simulink model "Praktikum02"  (R2023b)
settings: Solver=VariableStepAuto  StartTime=0.0  StopTime=10.0  RelTol=1e-3
model workspace (MAT data in the model file):
  M = 16
  Ts = 1e-06
undefined symbols (not defined in the file): doppler
libraries: commchan3 x8, commrflib2 x8, commdigbbndam3 x5, commsink2 x4, commrandsrc3 x1
settings Model: Creator=suttarar@hu-berlin.de

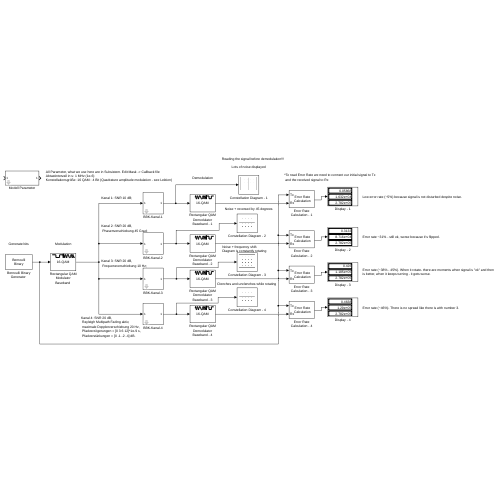
[thumbnail: Simulink's stored preview of the top-level diagram]
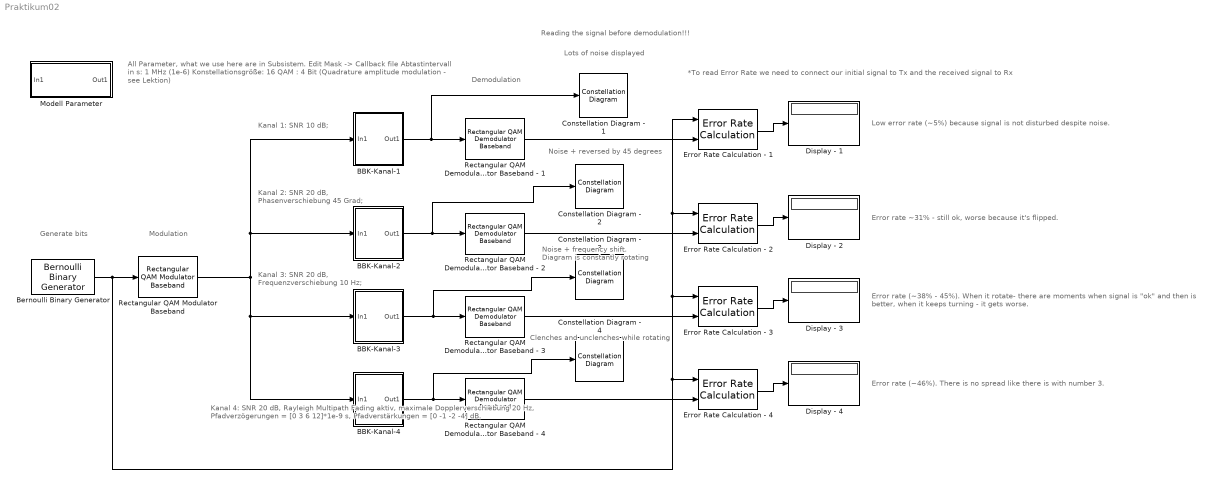
== system Praktikum02 ==
  note: Reading the signal before demodulation!!!
  note: *To read Error Rate we need to connect our initial signal to Tx
      |  and the received signal to Rx
  note: Error rate (~46%). There is no spread like there is with number 3.
  note: Clenches and unclenches while rotating
  note: Error rate (~38% - 45%). When it rotate- there are moments when signal is "ok" and then is better, when it keeps turning - it gets worse.
  note: Noise + frequency shift.
      | Diagram is constantly rotating
  note: Error rate ~31% - still ok, worse because it's flipped.
  note: Noise + reversed by 45 degrees
  note: Low error rate (~5%) because signal is not disturbed despite noise.
  note: Lots of noise displayed
  note: Kanal 4: SNR 20 dB,
      |  Rayleigh Multipath Fading aktiv,
      |  maximale Dopplerverschiebung 20 Hz,
      |  Pfadverzögerungen = [0 3 6 12]*1e-9 s,
      |  Pfadverstärkungen = [0 -1 -2 -4] dB.
  note: Kanal 3: SNR 20 dB,
      |  Frequenzverschiebung 10 Hz;
  note: Kanal 2: SNR 20 dB,
      |  Phasenverschiebung 45 Grad;
  note: Kanal 1: SNR 10 dB;
  note: Modulation
  note: Generate bits
  note: All Parameter, what we use here are in Subsistem. Edit Mask -> Callback file
      | Abtastintervall in s: 1 MHz (1e-6)
      | Konstellationsgröße: 16 QAM : 4 Bit (Quadrature amplitude modulation - see Lektion)
  note: Demodulation
  BBK-Kanal-1 : Subsystem  mask{MaxDoppler=20, PathDelays=[0 3 6 12]*1e-9, PathGains=[0 -1 -2 -4], EnableMultipath=0, PathLoss=0, FrequencyOffset=0, PhaseOffset=0, SNR=10}
      mask prompts: MaxDoppler "Dopplerverschiebung"; PathDelays "Pfadverzoergerungen"; PathGains "Pfadverstaerkungen"; EnableMultipath "SwitchBlock"; PathLoss "Pfadverlust"; FrequencyOffset "Frequenzverschiebung"; PhaseOffset "Phasenverschiebung"; SNR "AWG-Rauschen"
  BBK-Kanal-2 : Subsystem  mask{MaxDoppler=20, PathDelays=[0 3 6 12]*1e-9, PathGains=[0 -1 -2 -4], EnableMultipath=0, PathLoss=0, FrequencyOffset=0, PhaseOffset=45, SNR=20}
      mask prompts: MaxDoppler "Dopplerverschiebung"; PathDelays "Pfadverzoergerungen"; PathGains "Pfadverstaerkungen"; EnableMultipath "SwitchBlock"; PathLoss "Pfadverlust"; FrequencyOffset "Frequenzverschiebung"; PhaseOffset "Phasenverschiebung"; SNR "AWG-Rauschen"
  BBK-Kanal-3 : Subsystem  mask{MaxDoppler=20, PathDelays=[0 3 6 12]*1e-9, PathGains=[0 -1 -2 -4], EnableMultipath=0, PathLoss=0, FrequencyOffset=10, PhaseOffset=0, SNR=20}
      mask prompts: MaxDoppler "Dopplerverschiebung"; PathDelays "Pfadverzoergerungen"; PathGains "Pfadverstaerkungen"; EnableMultipath "SwitchBlock"; PathLoss "Pfadverlust"; FrequencyOffset "Frequenzverschiebung"; PhaseOffset "Phasenverschiebung"; SNR "AWG-Rauschen"
  BBK-Kanal-4 : Subsystem  mask{MaxDoppler=20, PathDelays=[0 3 6 12]*1e-9, PathGains=[0 -1 -2 -4], EnableMultipath=1, PathLoss=0, FrequencyOffset=0, PhaseOffset=0, SNR=20}
      mask prompts: MaxDoppler "Dopplerverschiebung"; PathDelays "Pfadverzoergerungen"; PathGains "Pfadverstaerkungen"; EnableMultipath "SwitchBlock"; PathLoss "Pfadverlust"; FrequencyOffset "Frequenzverschiebung"; PhaseOffset "Phasenverschiebung"; SNR "AWG-Rauschen"
  "Bernoulli Binary Generator " : commrandsrc3/Bernoulli Binary Generator  ProbabilityOfZero=0.5  SeedSource=Auto  Seed=0  SampleTime=Ts  SamplesPerFrame=log2(M)  OutputDataType=double  SimulateUsing=Interpreted execution
  Constellation Diagram - 1 : ConstellationDiagram  WindowPosition=[-8.000000,434.000000,600.000000,600.000000,]  Visible=on  ScopeFrameLocation=window  SymbolsToDisplaySource=Property  SymbolsToDisplay=500  XLimits=[-1.46,1.46]  YLimits=[-1.38,1.38]
  Constellation Diagram - 2 : ConstellationDiagram  WindowPosition=[602.000000,302.000000,600.000000,600.000000,]  Visible=on  ScopeFrameLocation=window  SymbolsToDisplaySource=Property  SymbolsToDisplay=500  ReferenceConstellation=QPSK  XLimits=[-1.46,1.46]  YLimits=[-1.38,1.38]
  Constellation Diagram - 3 : ConstellationDiagram  WindowPosition=[-15.000000,-148.000000,600.000000,600.000000,]  Visible=on  ScopeFrameLocation=window  SymbolsToDisplaySource=Property  SymbolsToDisplay=500  XLimits=[-1.46,1.46]  YLimits=[-1.38,1.38]
  Constellation Diagram - 4 : ConstellationDiagram  WindowPosition=[632.000000,-181.000000,600.000000,600.000000,]  Visible=on  ScopeFrameLocation=window  SymbolsToDisplaySource=Property  SymbolsToDisplay=500  XLimits=[-1.46,1.46]  YLimits=[-1.38,1.38]
  Display - {1..4} (4 alike) : Display
  Error Rate Calculation - {1..4} (4 alike) : commsink2/Error Rate Calculation  N=0  st_delay=0  cp_mode=Entire frame  subframe=[]  PMode=Port  WsName=ErrorVec  RsMode2=off  stop=off  numErr=100  maxBits=1e6
  Modell Parameter : Subsystem  mask{Ts=1e-6, M=16}
      mask prompts: Ts "Abtastintervall in s"; M "Konstellationsgröße"
  Rectangular QAM Demodulator Baseband - {1..4} (4 alike) : commdigbbndam3/Rectangular QAM Demodulator Baseband  M=M  OutType=Bit  DecType=Hard decision  VarSource=Dialog  Variance=1  Dec=Gray  Mapping=[0:15]  PowType=Average Power  MinDist=2  AvgPow=1  PeakPow=1  Ph=0  outDtype1=Inherit via internal rule  outDtype2=Inherit via internal rule  derotateFactorWordLen=16  derotateFactorDataTypeStr=Inherit: Same word length as input  derotateFactorLastDataTypeStr=Inherit: Same word length as input  denormFactorWordLen=16  denormFactorDataTypeStr=Inherit: Same word length as input  denormFactorLastDataTypeStr=Inherit: Same word length as input  prodOutWordLen=32  prodOutOverflowMode=Wrap  prodOutRoundingMode=Floor  prodOutOvFlMode=off  prodOutOvFlModeLastStrValue=off  sumWordLen=32
  "Rectangular QAM Modulator Baseband " : commdigbbndam3/Rectangular QAM Modulator Baseband  M=M  InType=Bit  Enc=Gray  Mapping=[0:15]  PowType=Average Power  MinDist=2  AvgPow=1  PeakPow=1  Ph=0  outDtype=double  outWordLen=16  outUDDataType=sfix(16)  outFracLenMode=Best precision  outFracLen=15  outDataTypeStr=double  outLastDataTypeStr=double
  wires:
  "Bernoulli Binary Generator "/1 -> Error Rate Calculation - 4/1, Error Rate Calculation - 3/1, Error Rate Calculation - 2/1, Error Rate Calculation - 1/1, "Rectangular QAM Modulator Baseband "/1
  "Rectangular QAM Modulator Baseband "/1 -> BBK-Kanal-1/1(In1), BBK-Kanal-2/1(In1), BBK-Kanal-4/1(In1), BBK-Kanal-3/1(In1)
  BBK-Kanal-1/1(Out1) -> Constellation Diagram - 1/1, Rectangular QAM Demodulator Baseband - 1/1
  BBK-Kanal-2/1(Out1) -> Constellation Diagram - 2/1, Rectangular QAM Demodulator Baseband - 2/1
  BBK-Kanal-3/1(Out1) -> Constellation Diagram - 3/1, Rectangular QAM Demodulator Baseband - 3/1
  BBK-Kanal-4/1(Out1) -> Constellation Diagram - 4/1, Rectangular QAM Demodulator Baseband - 4/1
  Error Rate Calculation - 1/1 -> Display - 1/1
  Error Rate Calculation - 2/1 -> Display - 2/1
  Error Rate Calculation - 3/1 -> Display - 3/1
  Error Rate Calculation - 4/1 -> Display - 4/1
  Rectangular QAM Demodulator Baseband - 4/1 -> Error Rate Calculation - 4/2
  Rectangular QAM Demodulator Baseband - 3/1 -> Error Rate Calculation - 3/2
  Rectangular QAM Demodulator Baseband - 2/1 -> Error Rate Calculation - 2/2
  Rectangular QAM Demodulator Baseband - 1/1 -> Error Rate Calculation - 1/2

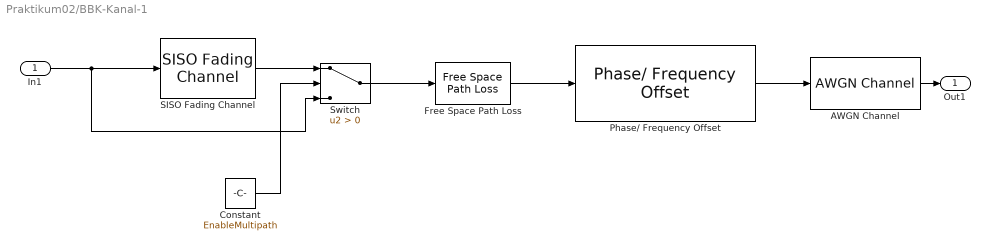
== system Praktikum02/BBK-Kanal-1 ==
  In1 : Inport
  AWGN Channel : commchan3/AWGN Channel  LegacyMode=off  NoiseMethod="Signal to noise ratio  (SNR)"  noiseMode="Signal to noise ratio  (SNR)"  EbNo=10  EsNo=10  SNR=SNR  BitsPerSymbol=1  SignalPower=1  SamplesPerSymbol=1  SymbolPeriod=1  VarianceSource=Parameter  Variance=1  RandomStream=Global stream  Seed=67  SimulateUsing=Code generation
  Constant : Constant  Value=EnableMultipath
  Free Space Path Loss : commrflib2/Free Space Path Loss  mode=Decibels  dB=PathLoss  d=0.100  fc=1920
  Phase/ Frequency Offset : commrflib2/Phase// Frequency Offset  phaseOffset=PhaseOffset  freqPort=off  freqOffset=FrequencyOffset
      settings: LibrarySourceBlock=|
      | commrfcorlib/Phase//
      | Frequency
      | Offset
  SISO Fading Channel : commchan3/SISO Fading Channel  InheritSampleRate=on  SampleRate=1  PathDelays=PathDelays  AveragePathGains=PathGains  NormalizePathGains=on  FadingDistribution=Rayleigh  KFactor=3  DirectPathDopplerShift=0  DirectPathInitialPhase=0  MaximumDopplerShift=MaxDoppler  DopplerSpectrum=doppler('Jakes')  RandomStream=mt19937ar with seed  Seed=73  PathGainsOutputPort=off  ChannelFilterDelayOutputPort=off  SimulateUsing=Interpreted execution  Visualization=Off  PathsForDopplerDisplay=1  SamplesToDisplay=25%
  Switch : Switch  Criteria=u2 > Threshold  SaturateOnIntegerOverflow=off  InputSameDT=off
  Out1 : Outport
  wires:
  Phase/ Frequency Offset/1 -> AWGN Channel/1
  Free Space Path Loss/1 -> Phase/ Frequency Offset/1
  AWGN Channel/1 -> Out1/1
  Switch/1 -> Free Space Path Loss/1
  SISO Fading Channel/1 -> Switch/1
  In1/1 -> Switch/3, SISO Fading Channel/1
  Constant/1 -> Switch/2

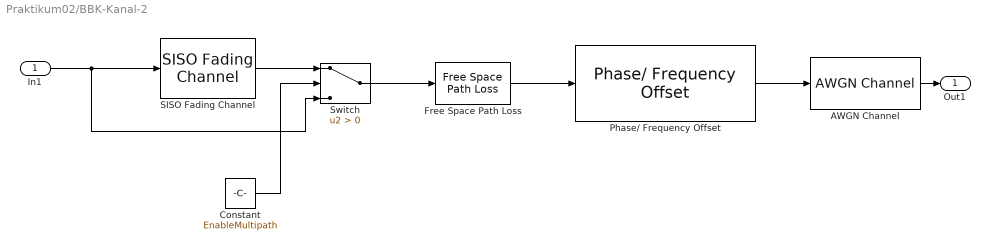
== system Praktikum02/BBK-Kanal-2 ==
  In1 : Inport
  AWGN Channel : commchan3/AWGN Channel  LegacyMode=off  NoiseMethod="Signal to noise ratio  (SNR)"  noiseMode="Signal to noise ratio  (SNR)"  EbNo=10  EsNo=10  SNR=SNR  BitsPerSymbol=1  SignalPower=1  SamplesPerSymbol=1  SymbolPeriod=1  VarianceSource=Parameter  Variance=1  RandomStream=Global stream  Seed=67  SimulateUsing=Code generation
  Constant : Constant  Value=EnableMultipath
  Free Space Path Loss : commrflib2/Free Space Path Loss  mode=Decibels  dB=PathLoss  d=0.100  fc=1920
  Phase/ Frequency Offset : commrflib2/Phase// Frequency Offset  phaseOffset=PhaseOffset  freqPort=off  freqOffset=FrequencyOffset
      settings: LibrarySourceBlock=|
      | commrfcorlib/Phase//
      | Frequency
      | Offset
  SISO Fading Channel : commchan3/SISO Fading Channel  InheritSampleRate=on  SampleRate=1  PathDelays=PathDelays  AveragePathGains=PathGains  NormalizePathGains=on  FadingDistribution=Rayleigh  KFactor=3  DirectPathDopplerShift=0  DirectPathInitialPhase=0  MaximumDopplerShift=MaxDoppler  DopplerSpectrum=doppler('Jakes')  RandomStream=mt19937ar with seed  Seed=73  PathGainsOutputPort=off  ChannelFilterDelayOutputPort=off  SimulateUsing=Interpreted execution  Visualization=Off  PathsForDopplerDisplay=1  SamplesToDisplay=25%
  Switch : Switch  Criteria=u2 > Threshold  SaturateOnIntegerOverflow=off  InputSameDT=off
  Out1 : Outport
  wires:
  Phase/ Frequency Offset/1 -> AWGN Channel/1
  Free Space Path Loss/1 -> Phase/ Frequency Offset/1
  AWGN Channel/1 -> Out1/1
  Switch/1 -> Free Space Path Loss/1
  SISO Fading Channel/1 -> Switch/1
  In1/1 -> Switch/3, SISO Fading Channel/1
  Constant/1 -> Switch/2

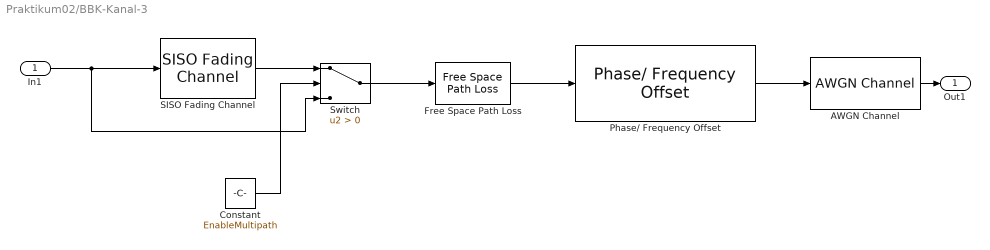
== system Praktikum02/BBK-Kanal-3 ==
  In1 : Inport
  AWGN Channel : commchan3/AWGN Channel  LegacyMode=off  NoiseMethod="Signal to noise ratio  (SNR)"  noiseMode="Signal to noise ratio  (SNR)"  EbNo=10  EsNo=10  SNR=SNR  BitsPerSymbol=1  SignalPower=1  SamplesPerSymbol=1  SymbolPeriod=1  VarianceSource=Parameter  Variance=1  RandomStream=Global stream  Seed=67  SimulateUsing=Code generation
  Constant : Constant  Value=EnableMultipath
  Free Space Path Loss : commrflib2/Free Space Path Loss  mode=Decibels  dB=PathLoss  d=0.100  fc=1920
  Phase/ Frequency Offset : commrflib2/Phase// Frequency Offset  phaseOffset=PhaseOffset  freqPort=off  freqOffset=FrequencyOffset
      settings: LibrarySourceBlock=|
      | commrfcorlib/Phase//
      | Frequency
      | Offset
  SISO Fading Channel : commchan3/SISO Fading Channel  InheritSampleRate=on  SampleRate=1  PathDelays=PathDelays  AveragePathGains=PathGains  NormalizePathGains=on  FadingDistribution=Rayleigh  KFactor=3  DirectPathDopplerShift=0  DirectPathInitialPhase=0  MaximumDopplerShift=MaxDoppler  DopplerSpectrum=doppler('Jakes')  RandomStream=mt19937ar with seed  Seed=73  PathGainsOutputPort=off  ChannelFilterDelayOutputPort=off  SimulateUsing=Interpreted execution  Visualization=Off  PathsForDopplerDisplay=1  SamplesToDisplay=25%
  Switch : Switch  Criteria=u2 > Threshold  SaturateOnIntegerOverflow=off  InputSameDT=off
  Out1 : Outport
  wires:
  Phase/ Frequency Offset/1 -> AWGN Channel/1
  Free Space Path Loss/1 -> Phase/ Frequency Offset/1
  AWGN Channel/1 -> Out1/1
  Switch/1 -> Free Space Path Loss/1
  SISO Fading Channel/1 -> Switch/1
  In1/1 -> Switch/3, SISO Fading Channel/1
  Constant/1 -> Switch/2

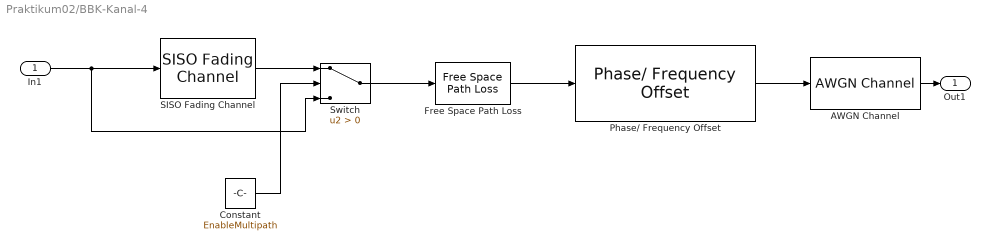
== system Praktikum02/BBK-Kanal-4 ==
  In1 : Inport
  AWGN Channel : commchan3/AWGN Channel  LegacyMode=off  NoiseMethod="Signal to noise ratio  (SNR)"  noiseMode="Signal to noise ratio  (SNR)"  EbNo=10  EsNo=10  SNR=SNR  BitsPerSymbol=1  SignalPower=1  SamplesPerSymbol=1  SymbolPeriod=1  VarianceSource=Parameter  Variance=1  RandomStream=Global stream  Seed=67  SimulateUsing=Code generation
  Constant : Constant  Value=EnableMultipath
  Free Space Path Loss : commrflib2/Free Space Path Loss  mode=Decibels  dB=PathLoss  d=0.100  fc=1920
  Phase/ Frequency Offset : commrflib2/Phase// Frequency Offset  phaseOffset=PhaseOffset  freqPort=off  freqOffset=FrequencyOffset
      settings: LibrarySourceBlock=|
      | commrfcorlib/Phase//
      | Frequency
      | Offset
  SISO Fading Channel : commchan3/SISO Fading Channel  InheritSampleRate=on  SampleRate=1  PathDelays=PathDelays  AveragePathGains=PathGains  NormalizePathGains=on  FadingDistribution=Rayleigh  KFactor=3  DirectPathDopplerShift=0  DirectPathInitialPhase=0  MaximumDopplerShift=MaxDoppler  DopplerSpectrum=doppler('Jakes')  RandomStream=mt19937ar with seed  Seed=73  PathGainsOutputPort=off  ChannelFilterDelayOutputPort=off  SimulateUsing=Interpreted execution  Visualization=Off  PathsForDopplerDisplay=1  SamplesToDisplay=25%
  Switch : Switch  Criteria=u2 > Threshold  SaturateOnIntegerOverflow=off  InputSameDT=off
  Out1 : Outport
  wires:
  Phase/ Frequency Offset/1 -> AWGN Channel/1
  Free Space Path Loss/1 -> Phase/ Frequency Offset/1
  AWGN Channel/1 -> Out1/1
  Switch/1 -> Free Space Path Loss/1
  SISO Fading Channel/1 -> Switch/1
  In1/1 -> Switch/3, SISO Fading Channel/1
  Constant/1 -> Switch/2

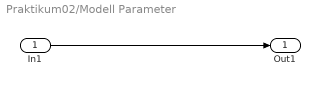
== system Praktikum02/Modell Parameter ==
  In1 : Inport
  Out1 : Outport
  wires:
  In1/1 -> Out1/1
